simulink model "Utkarsh_2005574_R_W2_P4"  (R2021a)
settings: Solver=ode45  StartTime=0.0  StopTime=0.08  RelTol=1e-3
PostLoadFcn:
  | J=3.2284e-6;
  | b=3.5077e-6;
  | K=0.0274;
  | R=4;
  | L=2.75e-6;
  | 
  | Kp=40.6275;
  | Ki=331.2128;
  | Kd=0.4934;
InitFcn:
  | J=3.2284e-6;
  | b=3.5077e-6;
  | K=0.0274;
  | R=4;
  | L=2.75e-6;
  | 
  | Kp=40.6275;
  | Ki=331.2128;
  | Kd=0.4934;
settings Model: Creator=Utkarsh Anand  LastModifiedBy=Utkarsh Anand

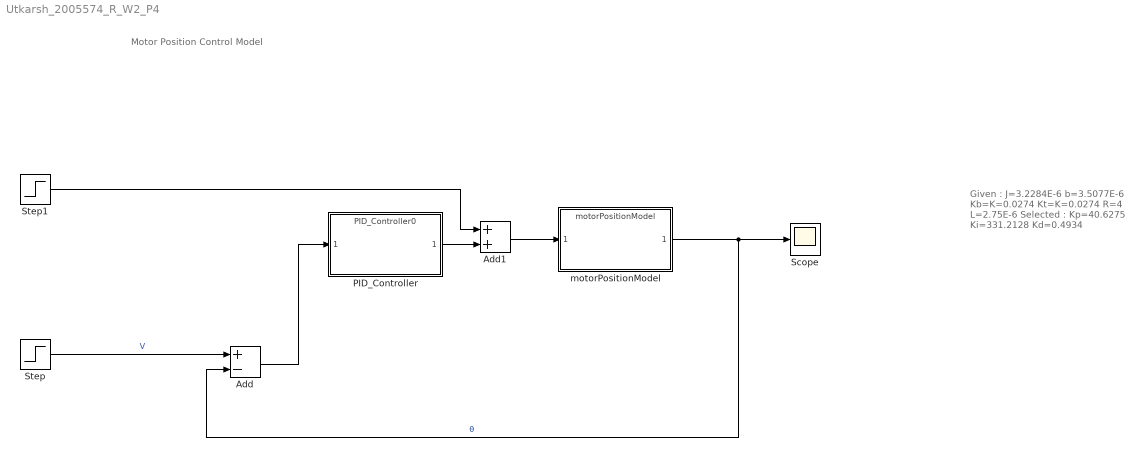
== system Utkarsh_2005574_R_W2_P4 ==
  note: Motor Position Control Model
  note: Given :
      | J=3.2284E-6
      | b=3.5077E-6
      | Kb=K=0.0274
      | Kt=K=0.0274
      | R=4
      | L=2.75E-6
      |
      | Selected :
      | Kp=40.6275
      | Ki=331.2128
      | Kd=0.4934
  Add : Sum  Inputs=+-
  Add1 : Sum
  PID_Controller : ModelReference  ModelNameDialog=PID_Controller0  SimulationMode=Normal  ModelReferenceVersion=1.7
  Scope : Scope
  Step : Step  Time=0  SampleTime=0
  Step1 : Step  Time=0.03  SampleTime=0
  motorPositionModel : ModelReference  ModelNameDialog=motorPositionModel  SimulationMode=Normal  ModelReferenceVersion=1.4
  wires:
  Step1/1 -> Add1/1
  Step/1 -> Add/1  "V"
  Add/1 -> PID_Controller/1
  PID_Controller/1 -> Add1/2
  Add1/1 -> motorPositionModel/1
  motorPositionModel/1 -> Add/2, Scope/1  "θ"
